simulink model "LQG_integratore"  (R2025b)
settings: Solver=VariableStepAuto  StartTime=0.0  StopTime=20.0  RelTol=1e-3
undefined symbols (not defined in the file): A, A_kf, B, B_kf, C, C_kf, D_kf, Kint1, Kint2, Qv, Rv
libraries: simulink x2
settings Model: Creator=inggi  LastModifiedBy=inggi

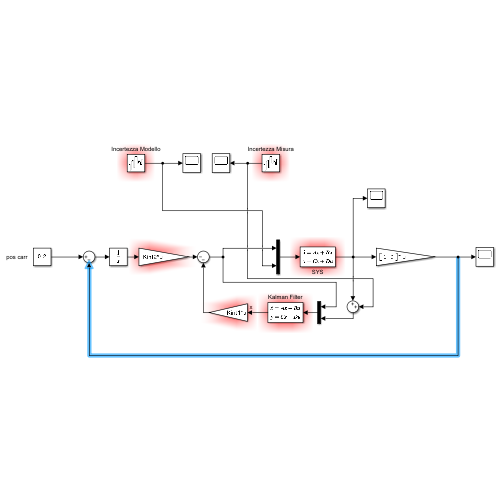
[thumbnail: Simulink's stored preview of the top-level diagram]
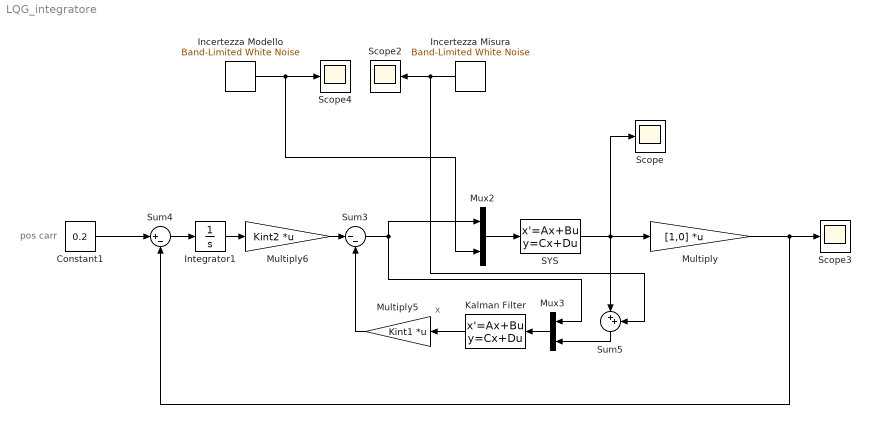
== system LQG_integratore ==
  note: x
  note: pos carr
  Constant1 : Constant  Value=0.2
  Incertezza Misura : simulink/Sources/Band-Limited White Noise  Cov=diag(Rv)  Ts=0.1  seed=[23341]
  Incertezza Modello : simulink/Sources/Band-Limited White Noise  Cov=diag(Qv)  Ts=0.1  seed=[23341]
  Integrator1 : Integrator
  Kalman Filter : StateSpace  A=A_kf  B=B_kf  C=C_kf  D=D_kf  InitialCondition=0
  Multiply : Gain  Gain=[1,0]  Multiplication=Matrix(K*u)
  Multiply5 : Gain  Gain=Kint1  Multiplication=Matrix(K*u)
  Multiply6 : Gain  Gain=Kint2  Multiplication=Matrix(K*u)
  Mux2 : Mux  Inputs=2
  Mux3 : Mux  Inputs=2
  SYS : StateSpace  A=A  B=[B, eye(4)]  C=C  D=zeros(2,5)  InitialCondition=0
  Scope{,2..4} (4 alike) : Scope
      Scope settings: ActiveDisplayYMinimum=-1  ActiveDisplayYMaximum=1
      Scope2 settings: DataLoggingVariableName=ScopeData2
      Scope3 settings: ActiveDisplayYMinimum=-0.02891780611158477  ActiveDisplayYMaximum=0.240431262661733  DataLoggingVariableName=ScopeData4
      Scope4 settings: DataLoggingVariableName=ScopeData3
  Sum3 : Sum  Inputs=|--
  Sum4 : Sum  Inputs=|+-
  Sum5 : Sum  Inputs=|++
  wires:
  Sum3/1 -> Mux2/1, Mux3/1
  Sum5/1 -> Mux3/2
  Multiply5/1 -> Sum3/2
  Mux3/1 -> Kalman Filter/1
  Multiply6/1 -> Sum3/1
  Sum4/1 -> Integrator1/1
  Constant1/1 -> Sum4/1
  Integrator1/1 -> Multiply6/1
  Kalman Filter/1 -> Multiply5/1
  Mux2/1 -> SYS/1
  Multiply/1 -> Sum4/2, Scope3/1
  SYS/1 -> Sum5/1, Scope/1, Multiply/1
  Incertezza Misura/1 -> Sum5/2, Scope2/1
  Incertezza Modello/1 -> Mux2/2, Scope4/1
